simulink model "VectorControl_Induction_motordrive"  (R2020a)
settings: Solver=ode45  StartTime=0  StopTime=1  MaxStep=Ts  RelTol=1e-3  AbsTol=1e-3  EnableMultiTasking=on
undefined symbols (not defined in the file or in its folder): alphac, alphas, J, LM, Lsigma, p, psiR_ref, RR, Rs, TM_max, Ts
libraries: simulink x2
settings Model: Creator=mhinkkan  LastModifiedBy=Dinesh Chandresh
settings SolverCC: AutoScaleAbsTol=off
settings DataIOCC: SaveFormat=Array  SignalLoggingSaveFormat=ModelDataLogs  SaveOutput=off  SignalLogging=off  DSMLogging=off  SaveTime=off  ReturnWorkspaceOutputs=off
settings OptimizationCC: BlockReduction=off  BooleanDataType=off  DefaultParameterBehavior=Inlined  OptimizeBlockIOStorage=off  BufferReuse=off  ExpressionFolding=off  ExpressionDepthLimit=2147483647  LocalBlockOutputs=off  InitFltsAndDblsToZero=on  LifeSpan=inf
settings DebuggingCC: SaveWithParameterizedLinksMsg=none  UnderspecifiedInitializationDetection=Classic  MergeDetectMultiDrivingBlocksExec=none  SignalResolutionControl=TryResolveAllWithWarning  MultiTaskDSMMsg=warning  MultiTaskCondExecSysMsg=none  FcnCallInpInsideContextMsg=warning  StateNameClashWarn=warning  SFUnexpectedBacktrackingDiag=warning  SFNoUnconditionalDefaultTransitionDiag=warning  SFExecutionAtInitializationDiag=none  ArithmeticOperatorsInVariantConditions=warning
settings HardwareCC: ProdBitPerPointer=32  ProdBitPerSizeT=32  ProdBitPerPtrDiffT=32  ProdLargestAtomicFloat=None  ProdIntDivRoundTo=Undefined  ProdEndianess=Unspecified  ProdWordSize=32  ProdHWDeviceType=32-bit Generic  TargetUnknown=on
settings ModelReferenceCC: PropagateSignalLabelsOutOfModel=off
settings SFSimCC: SimUseLocalCustomCode=off  CustomCodeUndefinedFunction=UseInterfaceOnly
settings RTWCC: RTWUseLocalCustomCode=off
settings CodeAppCC: StateflowObjectComments=on
settings GRTTargetCC: TargetFcnLib=ansi_tfl_tmw.mat  TargetLangStandard=C89/C90 (ANSI)  CombineOutputUpdateFcns=off  GRTInterface=on
settings ConfigComp: CovMetricSettings=dw  CovHtmlReporting=on  CovSaveCumulativeToWorkspaceVar=on  CovSaveSingleToWorkspaceVar=on  CovExternalEMLEnable=off

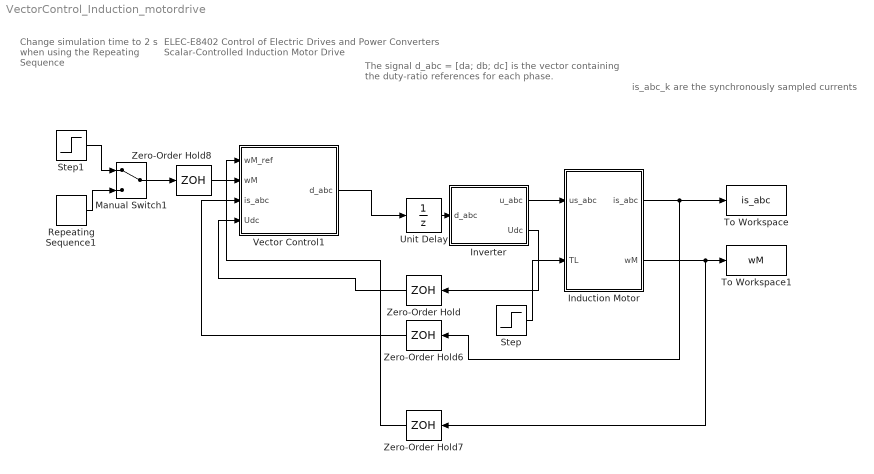
== system VectorControl_Induction_motordrive ==
  note: is_abc_k are the synchronously sampled currents
  note: The signal d_abc = [da; db; dc] is the vector
      | containing the duty-ratio references for each phase.
  note: ELEC-E8402 Control of Electric Drives and Power Converters
      |
      | Scalar-Controlled Induction Motor Drive
  note: Change simulation time
      | to 2 s when using the
      | Repeating Sequence
  Induction Motor : Subsystem  mask{Rs=3.7, RR=2.1, Lsigma=21e-3, LM=0.224, p=2, J=0.016}
      mask prompts: Rs "Stator resistance Rs (ohm)"; RR "Rotor resistance RR (ohm)"; Lsigma "Leakage inductance Lsigma (H)"; LM "Magnetizing inductance LM (H)"; p "Number of pole pairs p"; J "Total inertia J (kgm^2)"
      mask help: Inverse-Gamma model
  Inverter : Subsystem  mask{Ts=Ts, Udc=540}
      mask prompts: Ts "Sampling period Ts (s)"; Udc "DC-link voltage Udc (V)"
      mask help: The switching period is 2*Ts and the switching frequency is 1/(2*Ts).
  Manual Switch1 : ManualSwitch
  Repeating Sequence1 : simulink/Sources/Repeating Sequence  rep_seq_t=[0 .2 .8 1.2 1.8 2]  rep_seq_y=2*pi*30/p*[0 1 1 -1 -1 0]
  Step : Step  Time=.6  After=14.63  SampleTime=0
  Step1 : Step  Time=0.3  After=2*pi*40/p  SampleTime=Ts
  To Workspace : ToWorkspace  VariableName=is_abc  SaveFormat=Timeseries  SampleTime=-1
  To Workspace1 : ToWorkspace  VariableName=wM  SaveFormat=Timeseries  SampleTime=-1
  Unit Delay : UnitDelay  SampleTime=Ts  HasFrameUpgradeWarning=on
  Vector Control1 : Subsystem
  Zero-Order Hold{,6..8} (4 alike) : ZeroOrderHold  SampleTime=Ts
  wires:
  Step/1 -> Induction Motor/2(TL)
  Inverter/1(u_abc) -> Induction Motor/1(us_abc)
  Induction Motor/1(is_abc) -> Zero-Order Hold6/1, To Workspace/1
  Induction Motor/2(wM) -> Zero-Order Hold7/1, To Workspace1/1
  Manual Switch1/1 -> Zero-Order Hold8/1
  Step1/1 -> Manual Switch1/1
  Zero-Order Hold7/1 -> Vector Control1/2(wM)
  Zero-Order Hold/1 -> Vector Control1/4(Udc)
  Repeating Sequence1/1 -> Manual Switch1/2
  Vector Control1/1(d_abc) -> Unit Delay/1
  Zero-Order Hold6/1 -> Vector Control1/3(is_abc)
  Zero-Order Hold8/1 -> Vector Control1/1(wM_ref)
  Unit Delay/1 -> Inverter/1(d_abc)
  Inverter/2(Udc) -> Zero-Order Hold/1

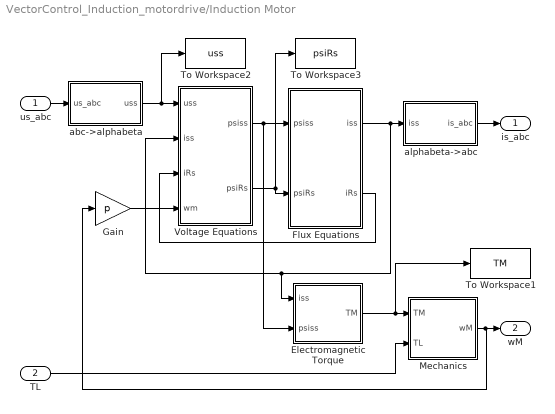
== system VectorControl_Induction_motordrive/Induction Motor ==
  us_abc : Inport
  TL : Inport  Port=2
  Electromagnetic Torque : Subsystem
  Flux Equations : Subsystem
  Gain : Gain  Gain=p  SaturateOnIntegerOverflow=on  OutDataTypeStr=Inherit: Same as input  ParamDataTypeStr=Inherit: Same as input
  Mechanics : Subsystem
  To Workspace1 : ToWorkspace  VariableName=TM  SaveFormat=Timeseries  SampleTime=-1
  To Workspace2 : ToWorkspace  VariableName=uss  SaveFormat=Timeseries  SampleTime=-1
  To Workspace3 : ToWorkspace  VariableName=psiRs  SaveFormat=Timeseries  SampleTime=-1
  Voltage Equations : Subsystem
  abc->alphabeta : Subsystem
  alphabeta->abc : Subsystem
  is_abc : Outport
  wM : Outport  Port=2
  wires:
  TL/1 -> Mechanics/2(TL)
  Mechanics/1(wM) -> wM/1, Gain/1
  Flux Equations/1(iss) -> Voltage Equations/2(iss), Electromagnetic Torque/1(iss), alphabeta->abc/1(iss)
  us_abc/1 -> abc->alphabeta/1(us_abc)
  Voltage Equations/2(psiRs) -> To Workspace3/1, Flux Equations/2(psiRs)
  Voltage Equations/1(psiss) -> Electromagnetic Torque/2(psiss), Flux Equations/1(psiss)
  Flux Equations/2(iRs) -> Voltage Equations/3(iRs)
  Electromagnetic Torque/1(TM) -> To Workspace1/1, Mechanics/1(TM)
  abc->alphabeta/1(uss) -> To Workspace2/1, Voltage Equations/1(uss)
  alphabeta->abc/1(is_abc) -> is_abc/1
  Gain/1 -> Voltage Equations/4(wm)

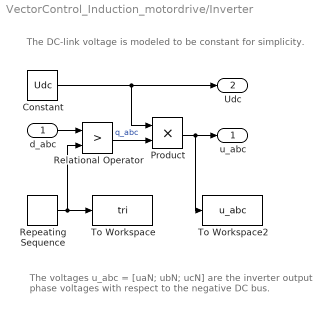
== system VectorControl_Induction_motordrive/Inverter ==
  note: The voltages u_abc = [uaN; ubN; ucN] are the inverter
      | output phase voltages with respect to the negative DC bus.
  note: The DC-link voltage is modeled to be constant for simplicity.
  d_abc : Inport
  Constant : Constant  Value=Udc  SampleTime=0
  Product : Product
  Relational Operator : RelationalOperator  Operator=>  OutDataTypeStr=boolean  RndMeth=Nearest
  Repeating Sequence : simulink/Sources/Repeating Sequence  rep_seq_t=[0 1 2]*Ts  rep_seq_y=[1 0 1]
  To Workspace : ToWorkspace  VariableName=tri  SaveFormat=Timeseries  SampleTime=-1
  To Workspace2 : ToWorkspace  VariableName=u_abc  SaveFormat=Timeseries  SampleTime=-1
  u_abc : Outport
  Udc : Outport  Port=2
  wires:
  Repeating Sequence/1 -> Relational Operator/2, To Workspace/1
  d_abc/1 -> Relational Operator/1
  Relational Operator/1 -> Product/2  "q_abc"
  Constant/1 -> Product/1, Udc/1
  Product/1 -> u_abc/1, To Workspace2/1

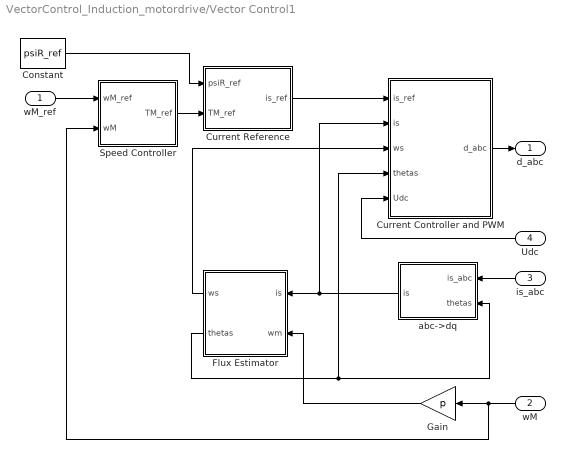
== system VectorControl_Induction_motordrive/Vector Control1 ==
  wM_ref : Inport
  wM : Inport  Port=2
  is_abc : Inport  Port=3
  Udc : Inport  Port=4
  Constant : Constant  Value=psiR_ref  SampleTime=Ts
  Current Controller and PWM : Subsystem
  Current Reference : Subsystem
  Flux Estimator : Subsystem
  Gain : Gain  Gain=p  SaturateOnIntegerOverflow=on  OutDataTypeStr=Inherit: Same as input  ParamDataTypeStr=Inherit: Same as input
  Speed Controller : Subsystem
  abc->dq : Subsystem
  d_abc : Outport
  wires:
  Flux Estimator/2(thetas) -> Current Controller and PWM/4(thetas), abc->dq/2(thetas)
  wM/1 -> Speed Controller/2(wM), Gain/1
  is_abc/1 -> abc->dq/1(is_abc)
  Current Controller and PWM/1(d_abc) -> d_abc/1
  Current Reference/1(is_ref) -> Current Controller and PWM/1(is_ref)
  Flux Estimator/1(ws) -> Current Controller and PWM/3(ws)
  abc->dq/1(is) -> Current Controller and PWM/2(is), Flux Estimator/1(is)
  wM_ref/1 -> Speed Controller/1(wM_ref)
  Constant/1 -> Current Reference/1(psiR_ref)
  Udc/1 -> Current Controller and PWM/5(Udc)
  Speed Controller/1(TM_ref) -> Current Reference/2(TM_ref)
  Gain/1 -> Flux Estimator/2(wm)

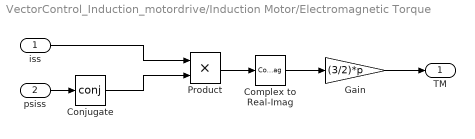
== system VectorControl_Induction_motordrive/Induction Motor/Electromagnetic Torque ==
  iss : Inport
  psiss : Inport  Port=2
  Complex to Real-Imag : ComplexToRealImag  Output=Imag
  Conjugate : Math  Operator=conj  SignedPower=on  RndMeth=Zero  SaturateOnIntegerOverflow=on
  Gain : Gain  Gain=(3/2)*p
  Product : Product
  TM : Outport
  wires:
  psiss/1 -> Conjugate/1
  Conjugate/1 -> Product/2
  iss/1 -> Product/1
  Gain/1 -> TM/1
  Product/1 -> Complex to Real-Imag/1
  Complex to Real-Imag/1 -> Gain/1

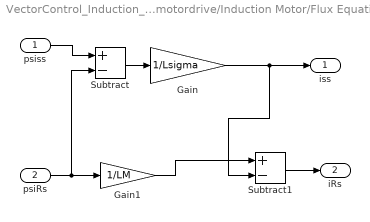
== system VectorControl_Induction_motordrive/Induction Motor/Flux Equations ==
  psiss : Inport
  psiRs : Inport  Port=2
  Gain : Gain  Gain=1/Lsigma
  Gain1 : Gain  Gain=1/LM
  Subtract : Sum  Inputs=+-
  Subtract1 : Sum  Inputs=+-
  iss : Outport
  iRs : Outport  Port=2
  wires:
  psiss/1 -> Subtract/1
  psiRs/1 -> Subtract/2, Gain1/1
  Subtract/1 -> Gain/1
  Gain/1 -> Subtract1/2, iss/1
  Gain1/1 -> Subtract1/1
  Subtract1/1 -> iRs/1

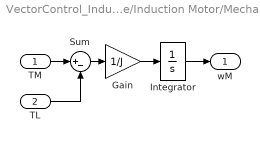
== system VectorControl_Induction_motordrive/Induction Motor/Mechanics ==
  TM : Inport
  TL : Inport  Port=2
  Gain : Gain  Gain=1/J  SaturateOnIntegerOverflow=on  OutDataTypeStr=Inherit: Same as input  ParamDataTypeStr=Inherit: Same as input
  Integrator : Integrator
  Sum : Sum  Inputs=|+-  InputSameDT=on  SaturateOnIntegerOverflow=on  OutDataTypeStr=Inherit: Same as first input
  wM : Outport
  wires:
  TL/1 -> Sum/2
  Sum/1 -> Gain/1
  Gain/1 -> Integrator/1
  Integrator/1 -> wM/1
  TM/1 -> Sum/1

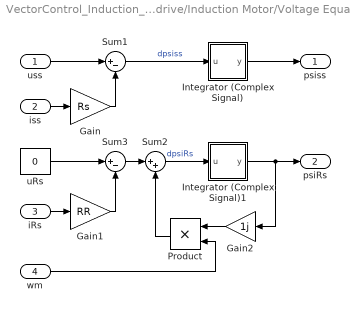
== system VectorControl_Induction_motordrive/Induction Motor/Voltage Equations ==
  uss : Inport
  iss : Inport  Port=2
  iRs : Inport  Port=3
  wm : Inport  Port=4
  Gain : Gain  Gain=Rs
  Gain1 : Gain  Gain=RR
  Gain2 : Gain  Gain=1j
  Integrator (Complex Signal) : Subsystem
      mask Display: disp('1/s');
  Integrator (Complex Signal)1 : Subsystem
      mask Display: disp('1/s');
  Product : Product  RndMeth=Zero
  Sum1 : Sum  Inputs=|+-
  Sum2 : Sum  Inputs=|++
  Sum3 : Sum  Inputs=|+-
  uRs : Constant  Value=0  SampleTime=0
  psiss : Outport
  psiRs : Outport  Port=2
  wires:
  uss/1 -> Sum1/1
  iss/1 -> Gain/1
  Sum1/1 -> Integrator (Complex Signal)/1(u)  "dpsiss"
  Gain/1 -> Sum1/2
  Integrator (Complex Signal)/1(y) -> psiss/1
  uRs/1 -> Sum3/1
  iRs/1 -> Gain1/1
  Gain1/1 -> Sum3/2
  Sum3/1 -> Sum2/1
  Sum2/1 -> Integrator (Complex Signal)1/1(u)  "dpsiRs"
  Product/1 -> Sum2/2
  Integrator (Complex Signal)1/1(y) -> psiRs/1, Gain2/1
  Gain2/1 -> Product/1
  wm/1 -> Product/2

== system VectorControl_Induction_motordrive/Induction Motor/abc->alphabeta ==
  us_abc : Inport
  Fcn : Fcn  Expr=2/3*(u(1)-0.5*u(2)-0.5*u(3))
  Fcn1 : Fcn  Expr=sqrt(3)/3*(u(2)-u(3))
  Real-Imag to Complex : RealImagToComplex
  uss : Outport
  wires:
  us_abc/1 -> Fcn1/1, Fcn/1
  Fcn/1 -> Real-Imag to Complex/1  "alpha"
  Fcn1/1 -> Real-Imag to Complex/2  "beta"
  Real-Imag to Complex/1 -> uss/1

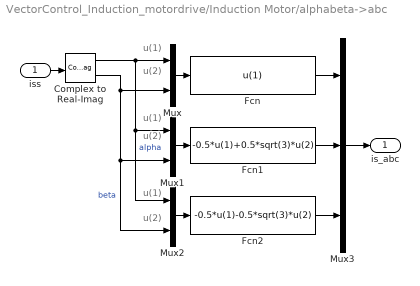
== system VectorControl_Induction_motordrive/Induction Motor/alphabeta->abc ==
  note: u(1)
  note: u(2)
  note: u(1)
  note: u(2)
  note: u(1)
  note: u(2)
  iss : Inport
  Complex to Real-Imag : ComplexToRealImag
  Fcn : Fcn  Expr=u(1)
  Fcn1 : Fcn  Expr=-0.5*u(1)+0.5*sqrt(3)*u(2)
  Fcn2 : Fcn  Expr=-0.5*u(1)-0.5*sqrt(3)*u(2)
  Mux : Mux  Inputs=2
  Mux1 : Mux  Inputs=2
  Mux2 : Mux  Inputs=2
  Mux3 : Mux  Inputs=3
  is_abc : Outport
  wires:
  Mux/1 -> Fcn/1
  Complex to Real-Imag/1 -> Mux/1, Mux1/1, Mux2/1  "alpha"
  Complex to Real-Imag/2 -> Mux/2, Mux1/2, Mux2/2  "beta"
  Mux1/1 -> Fcn1/1
  Mux2/1 -> Fcn2/1
  iss/1 -> Complex to Real-Imag/1
  Fcn/1 -> Mux3/1
  Fcn1/1 -> Mux3/2
  Fcn2/1 -> Mux3/3
  Mux3/1 -> is_abc/1

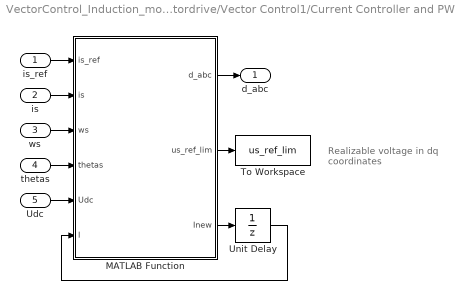
== system VectorControl_Induction_motordrive/Vector Control1/Current Controller and PWM ==
  note: Realizable voltage
      | in dq coordinates
  is_ref : Inport
  is : Inport  Port=2
  ws : Inport  Port=3
  thetas : Inport  Port=4
  Udc : Inport  Port=5
  MATLAB Function : MATLAB Function  TreatAsAtomicUnit=on
  To Workspace : ToWorkspace  VariableName=us_ref_lim  SaveFormat=Timeseries  SampleTime=-1
  Unit Delay : UnitDelay  SampleTime=-1  HasFrameUpgradeWarning=on
  d_abc : Outport  PortDimensions=3
  wires:
  MATLAB Function/3(Inew) -> Unit Delay/1
  is_ref/1 -> MATLAB Function/1(is_ref)
  ws/1 -> MATLAB Function/3(ws)
  is/1 -> MATLAB Function/2(is)
  Unit Delay/1 -> MATLAB Function/6(I)
  thetas/1 -> MATLAB Function/4(thetas)
  Udc/1 -> MATLAB Function/5(Udc)
  MATLAB Function/1(d_abc) -> d_abc/1
  MATLAB Function/2(us_ref_lim) -> To Workspace/1

== system VectorControl_Induction_motordrive/Vector Control1/Current Reference ==
  psiR_ref : Inport
  TM_ref : Inport  Port=2
  MATLAB Function : MATLAB Function  TreatAsAtomicUnit=on
  To Workspace2 : ToWorkspace  VariableName=is_ref  SaveFormat=Timeseries  SampleTime=-1
  is_ref : Outport
  wires:
  TM_ref/1 -> MATLAB Function/1(TM_ref)
  psiR_ref/1 -> MATLAB Function/2(psiR_ref)
  MATLAB Function/1(is_ref) -> To Workspace2/1, is_ref/1

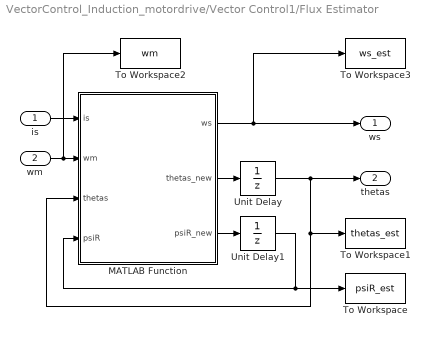
== system VectorControl_Induction_motordrive/Vector Control1/Flux Estimator ==
  is : Inport
  wm : Inport  Port=2
  MATLAB Function : MATLAB Function  TreatAsAtomicUnit=on
  To Workspace : ToWorkspace  VariableName=psiR_est  SaveFormat=Timeseries  SampleTime=-1
  To Workspace1 : ToWorkspace  VariableName=thetas_est  SaveFormat=Timeseries  SampleTime=-1
  To Workspace2 : ToWorkspace  VariableName=wm  SaveFormat=Timeseries  SampleTime=-1
  To Workspace3 : ToWorkspace  VariableName=ws_est  SaveFormat=Timeseries  SampleTime=-1
  Unit Delay : UnitDelay  SampleTime=-1  HasFrameUpgradeWarning=on
  Unit Delay1 : UnitDelay  SampleTime=-1  HasFrameUpgradeWarning=on
  ws : Outport
  thetas : Outport  Port=2
  wires:
  MATLAB Function/2(thetas_new) -> Unit Delay/1
  MATLAB Function/1(ws) -> To Workspace3/1, ws/1
  wm/1 -> To Workspace2/1, MATLAB Function/2(wm)
  is/1 -> MATLAB Function/1(is)
  Unit Delay1/1 -> MATLAB Function/4(psiR), To Workspace/1
  Unit Delay/1 -> MATLAB Function/3(thetas), To Workspace1/1, thetas/1
  MATLAB Function/3(psiR_new) -> Unit Delay1/1

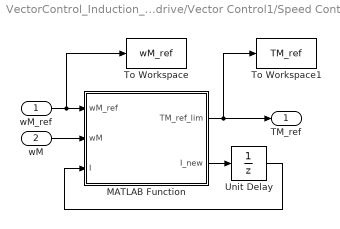
== system VectorControl_Induction_motordrive/Vector Control1/Speed Controller ==
  wM_ref : Inport
  wM : Inport  Port=2
  MATLAB Function : MATLAB Function  TreatAsAtomicUnit=on
  To Workspace : ToWorkspace  VariableName=wM_ref  SaveFormat=Timeseries  SampleTime=-1
  To Workspace1 : ToWorkspace  VariableName=TM_ref  SaveFormat=Timeseries  SampleTime=-1
  Unit Delay : UnitDelay  SampleTime=-1  HasFrameUpgradeWarning=on
  TM_ref : Outport
  wires:
  wM_ref/1 -> To Workspace/1, MATLAB Function/1(wM_ref)
  Unit Delay/1 -> MATLAB Function/3(I)
  wM/1 -> MATLAB Function/2(wM)
  MATLAB Function/1(TM_ref_lim) -> To Workspace1/1, TM_ref/1
  MATLAB Function/2(I_new) -> Unit Delay/1

== system VectorControl_Induction_motordrive/Vector Control1/abc->dq ==
  is_abc : Inport
  thetas : Inport  Port=2
  MATLAB Function : MATLAB Function  TreatAsAtomicUnit=on
  To Workspace4 : ToWorkspace  VariableName=is  SaveFormat=Timeseries  SampleTime=-1
  is : Outport
  wires:
  MATLAB Function/1(is) -> To Workspace4/1, is/1
  thetas/1 -> MATLAB Function/2(thetas)
  is_abc/1 -> MATLAB Function/1(is_abc)

== system VectorControl_Induction_motordrive/Induction Motor/Voltage Equations/Integrator (Complex Signal) ==
  u : Inport
  Complex to Real-Imag : ComplexToRealImag
  Integrator : Integrator
  Integrator1 : Integrator
  Real-Imag to Complex : RealImagToComplex
  y : Outport
  wires:
  Complex to Real-Imag/1 -> Integrator/1
  Complex to Real-Imag/2 -> Integrator1/1
  Integrator/1 -> Real-Imag to Complex/1
  Integrator1/1 -> Real-Imag to Complex/2
  Real-Imag to Complex/1 -> y/1
  u/1 -> Complex to Real-Imag/1

== system VectorControl_Induction_motordrive/Induction Motor/Voltage Equations/Integrator (Complex Signal)1 ==
  u : Inport
  Complex to Real-Imag : ComplexToRealImag
  Integrator : Integrator
  Integrator1 : Integrator
  Real-Imag to Complex : RealImagToComplex
  y : Outport
  wires:
  Complex to Real-Imag/1 -> Integrator/1
  Complex to Real-Imag/2 -> Integrator1/1
  Integrator/1 -> Real-Imag to Complex/1
  Integrator1/1 -> Real-Imag to Complex/2
  Real-Imag to Complex/1 -> y/1
  u/1 -> Complex to Real-Imag/1

== matlab function VectorControl_Induction_motordrive/Vector Control1/Current Controller and PWM/MATLAB Function ==
  data: is_ref input size=1; is input size=1; ws input size=1; thetas input size=1; Udc input size=1; I input size=1; Rs parameter size=1; Lsigma parameter size=1; alphac parameter size=1; Ts parameter size=1; d_abc output size=3; us_ref_lim output; Inew output
function [d_abc, us_ref_lim, Inew] = cc(is_ref, is, ws, thetas, Udc, I, Rs, Lsigma, alphac, Ts)
%#codegen

%% Current controller 
% Gains
kp = alphac*Lsigma;
ki = alphac^2*Lsigma;
Ra = alphac*Lsigma - Rs;

% Voltage reference in synchronous coordinates
e = is_ref - is;
us_ref = kp*e + ki*I - Ra*is + 1j*ws*Lsigma*is;

% Reference in stator coordinates
thetasc = thetas + 1.5*Ts*ws;   % Compensation for discrete-time delays
uss_ref = us_ref*exp(1j*thetasc);

%% Symmetrical suboscillation PWM
% Components of the voltage space vector
ualpha_ref = real(uss_ref);
ubeta_ref  = imag(uss_ref);

% Phase-voltage references
ua_ref = ualpha_ref;
ub_ref = .5*(-ualpha_ref + sqrt(3)*ubeta_ref);
uc_ref = .5*(-ualpha_ref - sqrt(3)*ubeta_ref);

% Vector of phase-voltage references
u_abc_ref = [ua_ref; ub_ref; uc_ref];

% Symmetrization of the references by adding the zero-sequence voltage
u0 = .5*(max(u_abc_ref) + min(u_abc_ref));
u_abc_ref = u_abc_ref - u0;

% Clamping of the reference voltages such that no phase error is caused. 
% If all phase voltage reference are realizable (below Udc/2), m = 1 holds.
m = max([2*u_abc_ref/Udc; 1]);
u_abc_ref = u_abc_ref/m;

% Duty cycles, which can be directly used for triangle comparison, 
% if the triangle wave varies between 0...1
d_abc = .5 + u_abc_ref/Udc;

% Realized voltage vector is calculated from the clamped duty ratios.
% If the PWM does not saturate, us_ref_lim = us_ref holds. The realized
% voltage vector is needed, e.g., for the current-controller antiwindup.
uss_ref_lim = 2/3*(d_abc(1) + d_abc(2)*exp(1j*2*pi/3) + d_abc(3)*exp(1j*4*pi/3))*Udc;
% In estimated rotor flux coordinates
us_ref_lim = exp(-1j*thetasc)*uss_ref_lim;  

%% Update the integral state of the current controller 
Inew = I + Ts*(e + (us_ref_lim - us_ref)/kp);

== matlab function VectorControl_Induction_motordrive/Vector Control1/Current Reference/MATLAB Function ==
  data: TM_ref input; psiR_ref input; LM parameter size=1; p parameter size=1; is_ref output
function is_ref = curr_ref(TM_ref, psiR_ref, LM, p)
%#codegen

% Current references in estimated rotor-flux coordinates
 id_ref =psiR_ref/LM;      
 iq_ref =(2*TM_ref)/(3*p*psiR_ref); 
is_ref = id_ref + 1j*iq_ref;

== matlab function VectorControl_Induction_motordrive/Vector Control1/Flux Estimator/MATLAB Function ==
  data: is input; wm input; thetas input; psiR input; RR parameter size=1; LM parameter size=1; Ts parameter size=1; ws output; thetas_new output; psiR_new output
function [ws, thetas_new, psiR_new] = estimator(is, wm, thetas, psiR, RR, LM, Ts)
%#codegen

% Current components
id = real(is);
iq = imag(is);

% Angular frequency of the rotor flux
if(psiR > 0)        % Avoid division by zero
    ws = wm + ((RR*iq)/psiR);      % Complete this
else
    ws = wm;
end

% Update the states
psiR_new = psiR+ Ts*RR*(id-(psiR/LM));                % Complete this
thetas_new = thetas + Ts*ws;    % Rotor flux angle

% Limit the angle between [-pi, pi]
while(thetas_new > pi)
    thetas_new = thetas_new - 2*pi;
end
while(thetas_new < -pi) 
    thetas_new = thetas_new + 2*pi;
end

== matlab function VectorControl_Induction_motordrive/Vector Control1/Speed Controller/MATLAB Function ==
  data: wM_ref input size=1; wM input size=1; I input size=1; J parameter size=1; alphas parameter size=1; TM_max parameter size=1; TM_ref_lim output size=1; Ts parameter size=1; I_new output
function [TM_ref_lim, I_new] = speed_ctrl(wM_ref, wM, I, J, alphas, TM_max, Ts)
%#codegen

% Speed controller
ba = alphas*J;
kp = alphas*J;
ki = alphas^2*J;

e = wM_ref - wM;
TM_ref = kp*e + ki*I - ba*wM;

% Limited reference
TM_ref_lim = TM_ref;
if(TM_ref_lim > TM_max)
    TM_ref_lim = TM_max;
elseif(TM_ref_lim < -TM_max)
    TM_ref_lim = -TM_max;
end

% Update state
I_new = I + Ts*(e + (TM_ref_lim - TM_ref)/kp);

== matlab function VectorControl_Induction_motordrive/Vector Control1/abc->dq/MATLAB Function ==
  data: is_abc input size=3; thetas input size=1; is output size=1
function is = abc_dq(is_abc, thetas)
%#codegen

% Phase currents
ia = is_abc(1); ib = is_abc(2); ic = is_abc(3); 

% Space-vector transformation and coordinate transformation
 is = (2/3)*(ia+(ib*exp((1j*2*pi)/3))+(ic*exp((1j*4*pi)/3)))*(exp(-1j*thetas));
